simulink model "encoder_arduino_test"  (R2021a)
settings: Solver=FixedStepAuto  StartTime=0.0  StopTime=inf  RelTol=1e-3  EnableMultiTasking=on
undefined symbols (not defined in the file): K3
libraries: arduinolib x3, eeGeneralControl x2
settings Model: SILPILModeSetting=veronly  ExtModeTrigDuration=2  Creator=mbelge  LastModifiedBy=youss
settings SolverCC: AlgebraicLoopSolver=TrustRegion
settings DataIOCC: LimitDataPoints=on  SaveFormat=Array  ReturnWorkspaceOutputs=off
settings OptimizationCC: EnhancedBackFolding=on  PassReuseOutputArgsAs=Individual arguments  ZeroExternalMemoryAtStartup=off  ZeroInternalMemoryAtStartup=off  MaxStackSize=64  OptimizeBlockOrder=speed  DifferentSizesBufferReuse=on  OptimizationCustomize=off  EfficientTunableParamExpr=on
settings DebuggingCC: UnderspecifiedInitializationDetection=Classic  MergeDetectMultiDrivingBlocksExec=none  ParameterTunabilityLossMsg=error  SFUnexpectedBacktrackingDiag=warning  SFNoUnconditionalDefaultTransitionDiag=warning  SFExecutionAtInitializationDiag=none  SFMachineParentedDataDiag=warning  ArithmeticOperatorsInVariantConditions=warning
settings HardwareCC: ProdBitPerInt=16  ProdBitPerPointer=16  ProdBitPerSizeT=16  ProdBitPerPtrDiffT=16  ProdLargestAtomicFloat=None  ProdWordSize=8  ProdHWDeviceType=Atmel->AVR
settings ModelReferenceCC: PropagateSignalLabelsOutOfModel=off
settings SFSimCC: SimUseLocalCustomCode=off  MATLABDynamicMemAlloc=off  CustomCodeUndefinedFunction=UseInterfaceOnly
settings RTWCC: SystemTargetFile=ert.tlc  HardwareBoard=Arduino Mega 2560  TemplateMakefile=ert_default_tmf  RTWVerbose=off  RTWUseLocalCustomCode=off  Toolchain=Arduino AVR  BuildConfiguration=Faster Runs
settings CodeAppCC: ForceParamTrailComments=on  IgnoreCustomStorageClasses=off  OperatorAnnotations=on  SimulinkDataObjDesc=on  SFDataObjDesc=on  InsertBlockDesc=on
settings ERTTargetCC: SupportContinuousTime=on  SupportVariableSizeSignals=on  ExtModeStaticAllocSize=2048
settings ConfigComp: CovMetricSettings=dw  CovSaveCumulativeToWorkspaceVar=on  CovSaveSingleToWorkspaceVar=on  CovExternalEMLEnable=off  CovSFcnEnable=off

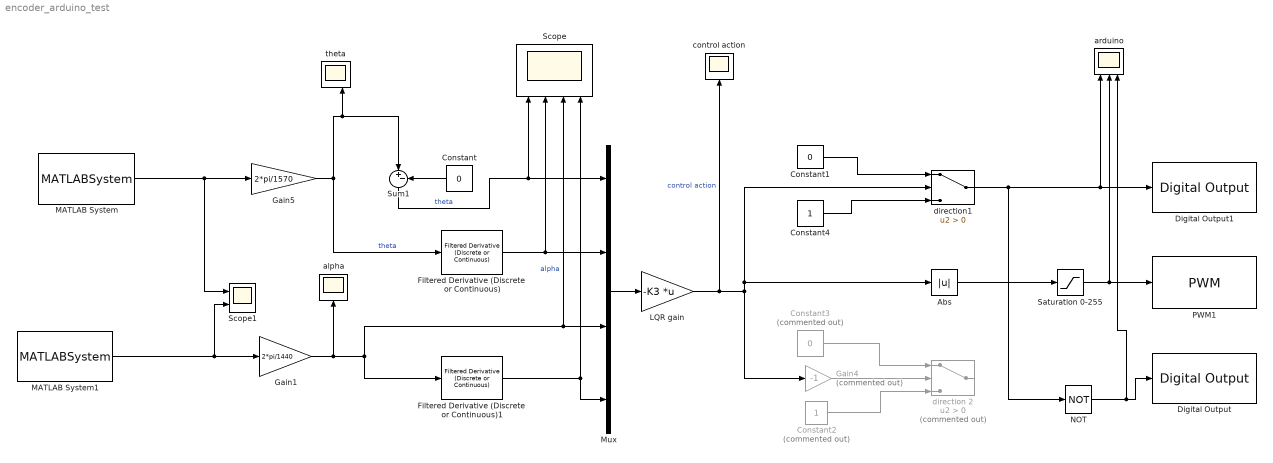
== system encoder_arduino_test ==
  Abs : Abs
  Constant : Constant  Value=0  SampleTime=-1
  Constant1 : Constant  Value=0
  Constant2 : Constant  Commented=on
  Constant3 : Constant  Commented=on  Value=0
  Constant4 : Constant
  Digital Output : arduinolib/Digital Output  pinNumber=8  Direction=output  blockPlatform=arduino
  Digital Output1 : arduinolib/Digital Output  pinNumber=7  Direction=output  blockPlatform=arduino
  Filtered Derivative (Discrete or Continuous) : eeGeneralControl/Filtered Derivative (Discrete or Continuous)  K=1  T=0.001  B=inf  A=-inf  minRatio=10  init_option=Inherited from block input  x0=0  Ts=-1
      settings: SourceProductBaseCode=PS
  Filtered Derivative (Discrete or Continuous)1 : eeGeneralControl/Filtered Derivative (Discrete or Continuous)  K=1  T=0.001  B=inf  A=-inf  minRatio=10  init_option=Inherited from block input  x0=0  Ts=-1
      settings: SourceProductBaseCode=PS
  Gain1 : Gain  Gain=2*pi/1440  OutDataTypeStr=double
  Gain4 : Gain  Commented=on  Gain=-1
  Gain5 : Gain  Gain=2*pi/1570  OutDataTypeStr=double
  "LQR gain " : Gain  Gain=-K3  Multiplication=Matrix(K*u)
  MATLAB System : MATLABSystem  System=Encoder_arduino  Encoder=0  PinA=19  PinB=18  SampleTime=0.001
      mask Type: Encoder_arduino
      mask Display:
      | disp('Encoder');
      | port_label('output',1,'y');
  MATLAB System1 : MATLABSystem  System=Encoder_arduino  Encoder=1  PinA=3  PinB=2  SampleTime=0.001
      mask Type: Encoder_arduino
      mask Display:
      | disp('Encoder');
      | port_label('output',1,'y');
  Mux : Mux
  NOT : Logic  Operator=NOT  IconShape=distinctive  AllPortsSameDT=off  OutDataTypeStr=boolean
  PWM1 : arduinolib/PWM  pinNumber=5  frequencyType=Default  desiredFrequency=490.2  achievableFrequency=490.2
  Saturation 0-255 : Saturate  UpperLimit=255  LowerLimit=80  LinearizeAsGain=off
      settings: LockScale=on
  Scope : Scope  NumInputPorts=4
  Scope1 : Scope  NumInputPorts=2
  Sum1 : Sum  Inputs=|+-
  alpha : Scope
  arduino : Scope  NumInputPorts=3
  "control action " : Scope
  direction 2 : Switch  Commented=on  Criteria=u2 > Threshold
  direction1 : Switch  Criteria=u2 > Threshold
  theta : Scope  NumInputPorts=2
  wires:
  Abs/1 -> Saturation 0-255/1
  Filtered Derivative (Discrete or Continuous)1/1 -> Mux/4, Scope/4
  Constant3/1 -> direction 2/1
  NOT/1 -> arduino/3, Digital Output/1
  MATLAB System1/1 -> Scope1/2, Gain1/1
  "LQR gain "/1 -> "control action "/1, direction1/2, Abs/1, Gain4/1  "control action"
  Saturation 0-255/1 -> arduino/2, PWM1/1
  MATLAB System/1 -> Scope1/1, Gain5/1
  Constant/1 -> Sum1/2
  Gain5/1 -> Sum1/1, theta/2, Filtered Derivative (Discrete or Continuous)/1  "theta"
  Constant1/1 -> direction1/1
  Sum1/1 -> Mux/1, Scope/1  "theta"
  direction1/1 -> NOT/1, arduino/1, Digital Output1/1
  Constant2/1 -> direction 2/3
  Mux/1 -> "LQR gain "/1
  Filtered Derivative (Discrete or Continuous)/1 -> Mux/2, Scope/2
  Constant4/1 -> direction1/3
  Gain4/1 -> direction 2/2
  Gain1/1 -> Mux/3, Scope/3, Filtered Derivative (Discrete or Continuous)1/1, alpha/1  "alpha"
